simulink model "MultiPortSwitch_3"  (R2017b)
settings: Solver=FixedStepDiscrete  StartTime=0.0  StopTime=10.0  FixedStep=0.200000  RelTol=1e-3
settings Model: Creator=hbourbou  LastModifiedBy=hbourbou
settings DataIOCC: SaveFormat=StructureWithTime
settings OptimizationCC: LifeSpan=inf
settings DebuggingCC: SFExecutionAtInitializationDiag=none
settings HardwareCC: ProdBitPerSizeT=32  ProdBitPerPtrDiffT=32  ProdWordSize=32  ProdHWDeviceType=Specified
settings CodeAppCC: StateflowObjectComments=on

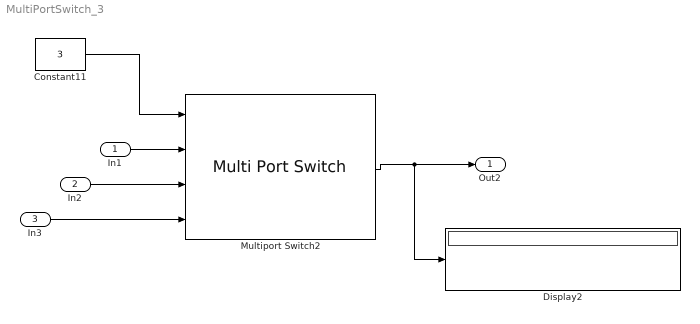
== system MultiPortSwitch_3 ==
  In1 : Inport  PortDimensions=[2,3]
  In2 : Inport  Port=2  PortDimensions=[2,3]
  In3 : Inport  Port=3  PortDimensions=[2,3]
  Constant11 : Constant  Value=3
  Display2 : Display
  Multiport Switch2 : MultiPortSwitch
  Out2 : Outport
  wires:
  Constant11/1 -> Multiport Switch2/1
  Multiport Switch2/1 -> Display2/1, Out2/1
  In1/1 -> Multiport Switch2/2
  In2/1 -> Multiport Switch2/3
  In3/1 -> Multiport Switch2/4
